simulink model "cruise_control_statefdbk"  (R2017a)
settings: Solver=VariableStepAuto  StartTime=0.0  StopTime=10.0  RelTol=1e-3
values from neighbouring files (symbols this model uses):
  damp = 50    [model.m]
  m = 1000    [model.m]
settings Model: Creator=Merc  LastModifiedBy=Merc

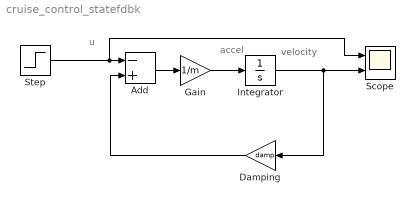
== system cruise_control_statefdbk ==
  note: u
  note: accel
  note: velocity
  Add : Sum  Inputs=-+
  "Damping " : Gain  Gain=damp
  Gain : Gain  Gain=1/m
  Integrator : Integrator  InitialCondition=1
  Scope : Scope  NumInputPorts=2
  Step : Step  After=0  SampleTime=0
  wires:
  Integrator/1 -> Scope/2, "Damping "/1
  "Damping "/1 -> Add/2
  Add/1 -> Gain/1
  Gain/1 -> Integrator/1
  Step/1 -> Scope/1, Add/1
